simulink model "simulinkmodelMissileGNC"  (R2025b)
settings: Solver=VariableStepAuto  StartTime=0.0  StopTime=10.0  RelTol=1e-3
values from neighbouring files (symbols this model uses):
  A = [-1.064 1.000; 290.26 0.00]    [model.m]
  B = [-0.25; -331.40]    [model.m]
  C = [-123.34 0.00; 0.00 1.00]    [model.m]
  D = [-13.51; 0]    [model.m]
  dT1 = 0.75    [model.m]
  dT2 = 0.25    [model.m]
  ELEV_INIT = 10000    [model.m]
  ELEV_TARGET = 795    [model.m]
  LAT_INIT = 34.2329    [model.m]
  LAT_OBS = 34.61916    [model.m]
  LAT_TARGET = 34.6588    [model.m]
  LON_INIT = -119.4573    [model.m]
  LON_OBS = -118.8429    [model.m]
  LON_TARGET = -118.769745    [model.m]
  Vel = 1021.08    [model.m]
undefined symbols (not defined in the file or in its folder): K, L
libraries: simulink x3, slpidlib x1
settings Model: Creator=vasis  LastModifiedBy=vasis

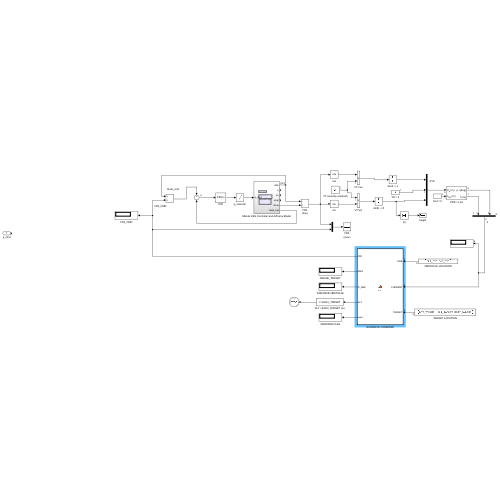
[thumbnail: Simulink's stored preview of the top-level diagram]
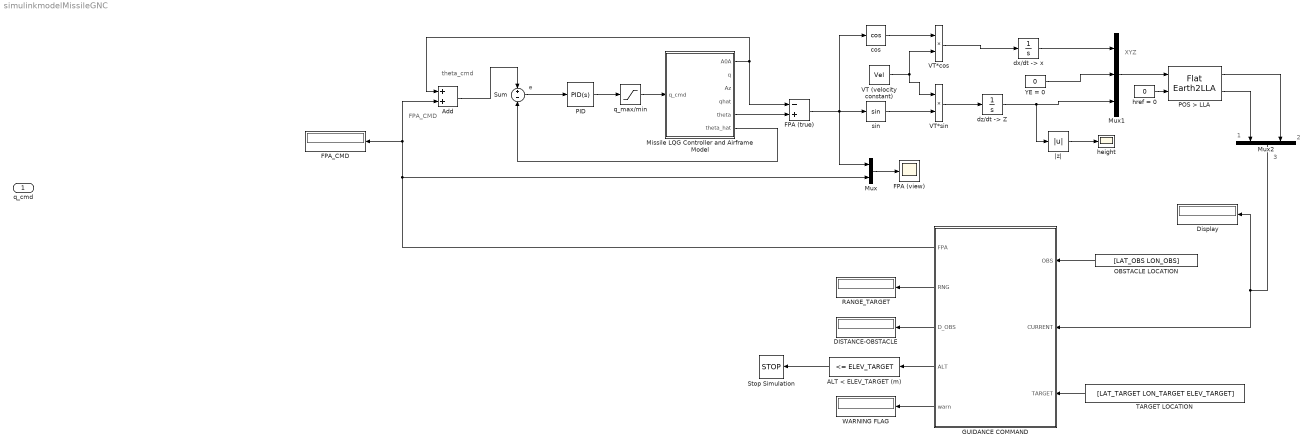
== system simulinkmodelMissileGNC ==
  note: 3
  note: 2
  note: 1
  note: XYZ
  note: theta_cmd
  note: FPA_CMD
  note: e
  q_cmd : Inport
  ALT < ELEV_TARGET (m) : simulink/Logic and Bit Operations/Compare To Constant  relop=<=  const=ELEV_TARGET  OutDataTypeStr=boolean
  Add : Sum
  DISTANCE-OBSTACLE : Display
  Display : Display
  FPA (true) : Sum  Inputs=-+
  FPA (view) : Scope
      settings: ActiveDisplayYMinimum=-30.70211204893462  ActiveDisplayYMaximum=4.2446791165482907
  FPA_CMD : Display
  GUIDANCE COMMAND : MATLAB Function  TreatAsAtomicUnit=on
  Missile LQG Controller and Airframe Model : Subsystem
  Mux : Mux  Inputs=2
  Mux1 : Mux  Inputs=3
  Mux2 : Mux  Inputs=2
  OBSTACLE LOCATION : Constant  Value=[LAT_OBS LON_OBS]
  PID : slpidlib/PID Controller  Controller=PID  Form=Parallel  TimeDomain=Continuous-time  UseExternalTs=off  SampleTime=-1  IntegratorMethod=Forward Euler  FilterMethod=Forward Euler  ControllerParametersSource=internal  P=-1  I=0  UseKiTs=off  D=0  UseExternalDerivativeSource=off  N=100  UseFilter=on  TunerSelectOption=Transfer Function Based (PID Tuner App)  InitialConditionSource=internal  InitialConditionForIntegrator=0  InitialConditionForFilter=0  DifferentiatorICPrevScaledInput=0  ExternalReset=none  TrackingMode=off  Kt=1  LimitOutput=off  SatLimitsSource=internal  UpperSaturationLimit=inf  LowerSaturationLimit=-inf  LinearizeAsGain=on  AntiWindupMode=none  Kb=1  LimitIntegrator=off  UpperIntegratorSaturationLimit=inf  LowerIntegratorSaturationLimit=-inf  POutMin=[]  POutMax=[]  IOutMin=[]  IOutMax=[]  DOutMin=[]  DOutMax=[]  NOutMin=[]  NOutMax=[]  SumOutMin=[]  SumOutMax=[]  SaturationOutMin=[]  SaturationOutMax=[]  PParamMin=[]  PParamMax=[]  IParamMin=[]  IParamMax=[]  DParamMin=[]  DParamMax=[]  NParamMin=[]  NParamMax=[]  KbParamMin=[]  KbParamMax=[]  KtParamMin=[]  KtParamMax=[]  KbOutMin=[]  KbOutMax=[]  KtOutMin=[]  KtOutMax=[]  IntegratorOutMin=[]  IntegratorOutMax=[]  FilterOutMin=[]  FilterOutMax=[]  SumI1OutMin=[]  SumI1OutMax=[]  SumI2OutMin=[]  SumI2OutMax=[]  SumI3OutMin=[]  SumI3OutMax=[]  SumI4OutMin=[]  SumI4OutMax=[]  SumDOutMin=[]  SumDOutMax=[]  DifferentiatorOutMin=[]  DifferentiatorOutMax=[]  FilterDiffOutCoefMin=[]  FilterDiffOutCoefMax=[]  ReciprocalOutMin=[]  ReciprocalOutMax=[]  SumDenOutMin=[]  SumDenOutMax=[]  SumNumOutMin=[]  SumNumOutMax=[]  DivideOutMin=[]  DivideOutMax=[]  UdiffTsProdOutMin=[]  UdiffTsProdOutMax=[]  NTsProdOutMin=[]  NTsProdOutMax=[]  UintegralTsProdOutMin=[]  UintegralTsProdOutMax=[]  UngainTsProdOutMin=[]  UngainTsProdOutMax=[]  ClampingZeroOutDataTypeStr=Inherit: Inherit via back propagation  ClampingZeroOutMin=[]  ClampingZeroOutMax=[]  FilterDenConstantOutDataTypeStr=Inherit: Inherit via back propagation  FilterDenConstantOutMin=[]  FilterDenConstantOutMax=[]  PCopyOutDataTypeStr=Inherit: Inherit via back propagation  PCopyOutMin=[]  PCopyOutMax=[]  NCopyOutDataTypeStr=Inherit: Inherit via back propagation  NCopyOutMin=[]  NCopyOutMax=[]  IntegratorContinuousStateAttributes=''  IntegratorStateMustResolveToSignalObject=off  IntegratorRTWStateStorageClass=Auto  FilterContinuousStateAttributes=''  FilterStateMustResolveToSignalObject=off  FilterRTWStateStorageClass=Auto  ParallelPVariant=InternalParameters  IdealPVariant=Disabled  IVariant=InternalParameters  DVariant=InternalParameters  IntegratorVariant=Continuous  SatVariant=Disabled  AWVariant=Passthrough  PCopyVariant=Disabled  TRVariant=Disabled  FdbkBlocksVariant=Forward  IdealPFdbkVariant=Disabled  SatFdbkVariant=Disabled  DerivativeFilterVariant=ContFilter  NVariant=InternalParameters  NCopyVariant=Disabled  FilterICVariant=InternalICsFilter  IntegratorICVariant=InternalICs  ExternalResetVariant=Disabled  TRSumVariant=Passthrough  SumFdbkVariant=Disabled  SumVariant=Sum_PID  TsampFilterVariant=InternalTs  TsampNgainVariant=Passthrough  TsampIntegralVariant=Disabled_SignalSpec  ExternalSaturationOutDataTypeStr=Inherit: Same as second input  DerivativeSourceVariant=ErrorSignal  PreIntVariant=InternalPreInt
  POS > LLA : FlatEarth2LLA  LL0=[LAT_INIT LON_INIT]  psi=yaw_init
  RANGE_TARGET : Display
  Stop Simulation : Stop
  Sum : Sum  Inputs=+-
  TARGET LOCATION : Constant  Value=[LAT_TARGET LON_TARGET ELEV_TARGET]
  VT (velocity constant) : Constant  Value=Vel
  VT*cos : Product
  VT*sin : Product
  WARNING FLAG : Display
  YE = 0 : Constant  Value=0
  cos : Trigonometry  Operator=cos
  "dx/dt -> x" : Integrator
  "dz/dt -> Z" : Integrator  InitialCondition=-ELEV_INIT
  height : Scope
      settings: DataLoggingVariableName=ScopeData2
  href = 0 : Constant  Value=0
  q_max/min : Saturate
  sin : Trigonometry
  |z| : Abs  SaturateOnIntegerOverflow=off
  wires:
  Missile LQG Controller and Airframe Model/1(A0A) -> Add/1, FPA (true)/1
  Missile LQG Controller and Airframe Model/5(theta) -> FPA (true)/2
  Missile LQG Controller and Airframe Model/6(theta_hat) -> Sum/2
  Add/1 -> Sum/1
  Sum/1 -> PID/1
  PID/1 -> q_max/min/1
  q_max/min/1 -> Missile LQG Controller and Airframe Model/1(q_cmd)
  Mux/1 -> FPA (view)/1
  FPA (true)/1 -> cos/1, Mux/1, sin/1
  sin/1 -> VT*sin/2
  cos/1 -> VT*cos/1
  VT (velocity constant)/1 -> VT*sin/1, VT*cos/2
  VT*cos/1 -> "dx/dt -> x"/1
  VT*sin/1 -> "dz/dt -> Z"/1
  YE = 0/1 -> Mux1/2
  "dx/dt -> x"/1 -> Mux1/1
  "dz/dt -> Z"/1 -> |z|/1, Mux1/3
  |z|/1 -> height/1
  Mux1/1 -> POS > LLA/1
  href = 0/1 -> POS > LLA/2
  POS > LLA/2 -> Mux2/1
  POS > LLA/1 -> Mux2/2
  OBSTACLE LOCATION/1 -> GUIDANCE COMMAND/1(OBS)
  TARGET LOCATION/1 -> GUIDANCE COMMAND/3(TARGET)
  Mux2/1 -> Display/1, GUIDANCE COMMAND/2(CURRENT)
  GUIDANCE COMMAND/3(D_OBS) -> DISTANCE-OBSTACLE/1
  GUIDANCE COMMAND/2(RNG) -> RANGE_TARGET/1
  GUIDANCE COMMAND/5(warn) -> WARNING FLAG/1
  GUIDANCE COMMAND/4(ALT) -> ALT < ELEV_TARGET (m)/1
  ALT < ELEV_TARGET (m)/1 -> Stop Simulation/1
  GUIDANCE COMMAND/1(FPA) -> Mux/2, Add/2, FPA_CMD/1

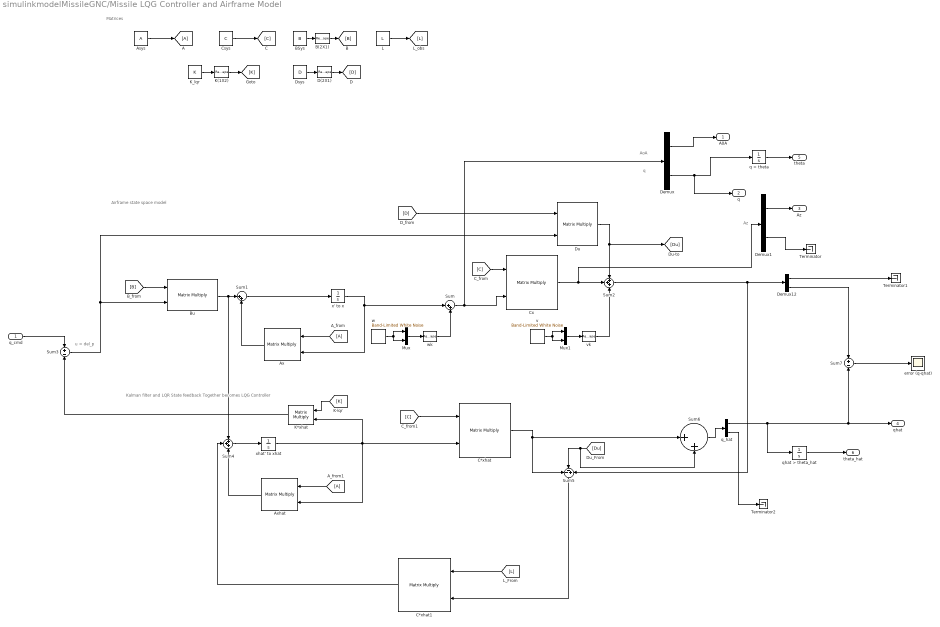
== system simulinkmodelMissileGNC/Missile LQG Controller and Airframe Model ==
  note: Az
  note: q
  note: AoA
  note: Kalman filter and LQR State feedback
      | Together becomes LQG Controller
  note: Airframe state space model
  note: u = del_p
  note: Matrices
  q_cmd : Inport
  A : Goto
  A_from : From
  A_from1 : From
  Asys : Constant  Value=A
  Ax : Product  Multiplication=Matrix(*)
  Axhat : Product  Multiplication=Matrix(*)
  B(2X1) : Reshape  OutputDimensionality=Customize  OutputDimensions=[2,1]
  BSys : Constant  Value=B
  Bu : Product  Multiplication=Matrix(*)
  C*xhat : Product  Multiplication=Matrix(*)
  C*xhat1 : Product  Multiplication=Matrix(*)
  Csys : Constant  Value=C
  Cx : Product  Multiplication=Matrix(*)
  D(2X1) : Reshape  OutputDimensionality=Customize  OutputDimensions=[2,1]
  Demux : Demux  Outputs=2
  Demux1 : Demux  Outputs=2
  Demux12 : Demux  Outputs=2
  Dsys : Constant  Value=D
  Du : Product  Multiplication=Matrix(*)
  K(1X2) : Reshape  OutputDimensionality=Customize  OutputDimensions=[1,2]
  K*xhat : Product  Multiplication=Matrix(*)
  K_lqr : Constant  Value=K
  L : Constant  Value=L
  Mux : Mux  Inputs=2
  Mux1 : Mux  Inputs=2
  Sum : Sum  Inputs=|++
  Sum1 : Sum  Inputs=|++
  Sum2 : Sum  Inputs=+++
  Sum3 : Sum  Inputs=+-
  Sum4 : Sum  Inputs=+++
  Sum5 : Sum  Inputs=--+
  Sum6 : Sum  Inputs=|++
  Sum7 : Sum  Inputs=+-
  Terminator : Terminator
  Terminator1 : Terminator
  Terminator2 : Terminator
  error (q-qhat) : Scope
  "q > theta " : Integrator
  q_hat : Demux  Outputs=2
  qhat > theta_hat : Integrator
  v : simulink/Sources/Band-Limited White Noise  Cov=[0.00001]  Ts=dT2  seed=[23341]
  vk : Reshape
  w : simulink/Sources/Band-Limited White Noise  Cov=[0.1]  Ts=dT1  seed=[23341]
  wk : Reshape  OutputDimensionality=Customize  OutputDimensions=[2,1]
  x' to x : Integrator
  xhat' to xhat : Integrator
  A0A : Outport
  q : Outport  Port=2
  Az : Outport  Port=3
  qhat : Outport  Port=4
  theta : Outport  Port=5
  theta_hat : Outport  Port=6
  wires:
  Sum3/1 -> Du/2, Bu/2
  vk/1 -> Sum2/3
  v/1 -> Mux1/1, Mux1/2
  L/1 -> [L]
  Sum5/1 -> C*xhat1/2
  Sum1/1 -> x' to x/1
  Sum4/1 -> xhat' to xhat/1
  K(1X2)/1 -> [K]
  Demux12/2 -> Sum7/1
  C*xhat/1 -> Sum5/1, Sum6/1
  Du/1 -> Sum2/1, [Du]
  K_lqr/1 -> K(1X2)/1
  x' to x/1 -> Sum/1, Ax/2
  Bu/1 -> Sum1/1, Sum4/1
  [K] -> K*xhat/1
  [Du] -> Sum6/2, Sum5/2
  Sum2/1 -> Demux12/1, Sum5/3
  C*xhat1/1 -> Sum4/2
  Sum/1 -> Demux/1, Cx/2
  Demux/2 -> q/1, "q > theta "/1
  [C] -> Cx/1
  Axhat/1 -> Sum4/3
  wk/1 -> Sum/2
  Demux/1 -> A0A/1
  [B] -> Bu/1
  [C] -> C*xhat/1
  qhat > theta_hat/1 -> theta_hat/1
  q_cmd/1 -> Sum3/1
  Sum6/1 -> q_hat/1
  Mux/1 -> wk/1
  K*xhat/1 -> Sum3/2
  w/1 -> Mux/1, Mux/2
  xhat' to xhat/1 -> K*xhat/2, Axhat/2, C*xhat/2
  [D] -> Du/1
  Cx/1 -> Demux1/1, Sum2/2
  Csys/1 -> [C]
  Asys/1 -> A/1
  A_from/1 -> Ax/1
  Sum7/1 -> error (q-qhat)/1
  BSys/1 -> B(2X1)/1
  Ax/1 -> Sum1/2
  Demux1/2 -> Terminator/1
  Demux12/1 -> Terminator1/1
  q_hat/1 -> qhat > theta_hat/1, qhat/1, Sum7/2
  B(2X1)/1 -> [B]
  A_from1/1 -> Axhat/1
  Mux1/1 -> vk/1
  [L] -> C*xhat1/1
  D(2X1)/1 -> [D]
  q_hat/2 -> Terminator2/1
  Dsys/1 -> D(2X1)/1
  "q > theta "/1 -> theta/1
  Demux1/1 -> Az/1

== matlab function simulinkmodelMissileGNC/GUIDANCE COMMAND ==
  data: OBS input; FPA output; CURRENT input; TARGET input; RNG output; D_OBS output; ALT output; warn output
function [FPA,RNG,D_OBS,ALT,warn] = fcn(OBS, CURRENT, TARGET)
%#codegen

R = 6.371e3;
d2r = pi/180;

%obstacle location
LAT_OBS = OBS(1);
LON_OBS = OBS(2);

%obstacle threshold (zone)
thres = 2000; %2km

%target location
LAT_TARGET = TARGET(1);
LON_TARGET = TARGET(2);
ELEV_TARGET = TARGET(3);

%CURRENT LOCATION
ELEV_CUR = CURRENT(1);
LAT_CUR = CURRENT(2);
LON_CUR = CURRENT(3);

%%DISTYANCE TO TARGET
l1 = LAT_CUR*d2r;
u1 = LON_CUR*d2r;
l2 = LAT_TARGET*d2r;
u2 = LON_TARGET*d2r;
dh = abs(ELEV_TARGET-ELEV_CUR);

dl = l2-l1;
du = u2-u1;

a = sin(dl/2)^2 + cos(l1)*cos(l2)*sin(du/2)^2;
c = 2*atan2(sqrt(a),sqrt(1-a));
d = R*c; %horizontal distance (in m)


%% DISTANCE FORM THE OBSTACLE
l3 = LAT_OBS*d2r;
u3 = LON_OBS*d2r;

dl = l3-l1;
du = u3-u1;

a = sin(dl/2)^2 + cos(l1)*cos(l2)*sin(du/2)^2;
c = 2*atan2(sqrt(a),sqrt(1-a));
d = R*c; %horizontal distance (in m)

%%CURRENT RANGE (FROM TARGET) - RANGE > DISTANCE

range = sqrt(d^2+dh^2);

%% calculate commanded fkight paht setpoint based on d_obs, range

if abs(d_obs)>=thres
    w = 0;
    FPA_CMD = atan(dh=d);
else
    %when in the obstacle zone, trigger warning
    w = 1;
    FPA_CMD = 0;
end

%%output variables


FPA = FPA_CMD;
RNG = range;
D_OBS = d_obs;
warn = w;
ALT = ELEV_CUR;


y = u;
